simulink model "task_1_simm"  (R2023a)
settings: Solver=VariableStepAuto  StartTime=0.0  StopTime=10.0  RelTol=1e-3
undefined symbols (not defined in the file): A, B, K, x0
settings Model: Creator=user  LastModifiedBy=user

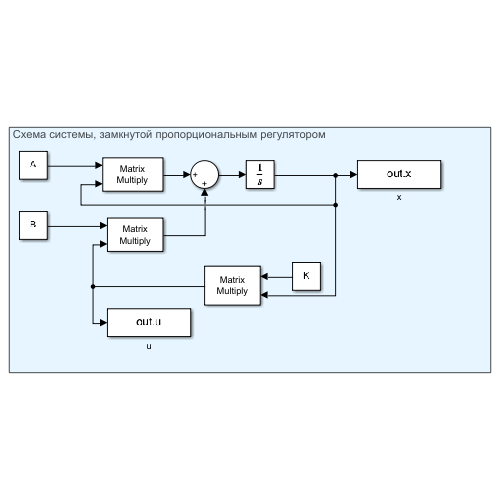
[thumbnail: Simulink's stored preview of the top-level diagram]
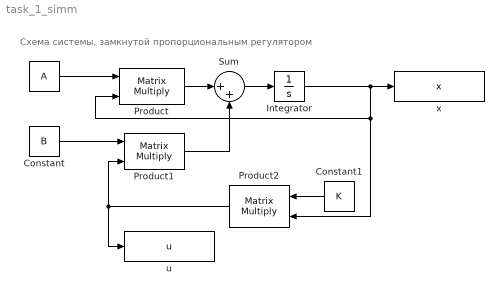
== system task_1_simm ==
  note: Схема системы, замкнутой пропорциональным регулятором
  " " : Constant  Value=A
  Constant : Constant  Value=B  VectorParams1D=off
  Constant1 : Constant  Value=K  VectorParams1D=off
  Integrator : Integrator  InitialCondition=x0
  Product : Product  Multiplication=Matrix(*)
  Product1 : Product  Multiplication=Matrix(*)
  Product2 : Product  Multiplication=Matrix(*)
  Sum : Sum  Inputs=|++
  u : ToWorkspace  VariableName=u  SaveFormat=Timeseries  SampleTime=-1
  x : ToWorkspace  VariableName=x  SaveFormat=Timeseries  SampleTime=-1
  wires:
  Product2/1 -> u/1, Product1/2
  Product/1 -> Sum/1
  Integrator/1 -> Product2/2, Product/2, x/1
  Sum/1 -> Integrator/1
  Constant/1 -> Product1/1
  " "/1 -> Product/1
  Product1/1 -> Sum/2
  Constant1/1 -> Product2/1
